simulink model "final_system"  (R2022b)
settings: Solver=FixedStepAuto  StartTime=0.0  StopTime=140  FixedStep=0.01  RelTol=1e-3
undefined symbols (not defined in the file or in its folder): heading_gain, omega0
libraries: SignalEditorBlockLib x1
settings Model: Creator=zd012  LastModifiedBy=zd012
settings DebuggingCC: UnconnectedInputMsg=warning  UnconnectedOutputMsg=warning  UnconnectedLineMsg=warning
settings ModelReferenceCC: EnableRefExpFcnMdlSchedulingChecks=on
settings RTWCC: DLArmComputeVersion=19.05

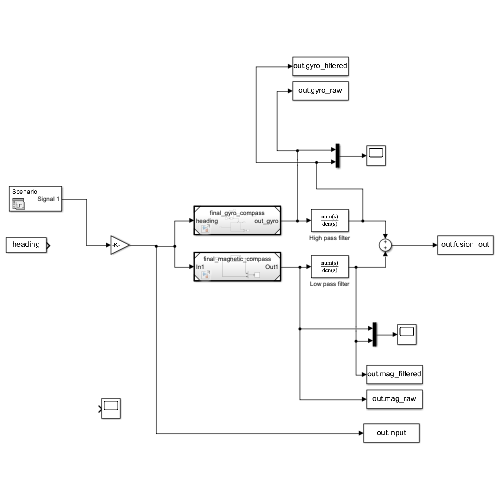
[thumbnail: Simulink's stored preview of the top-level diagram]
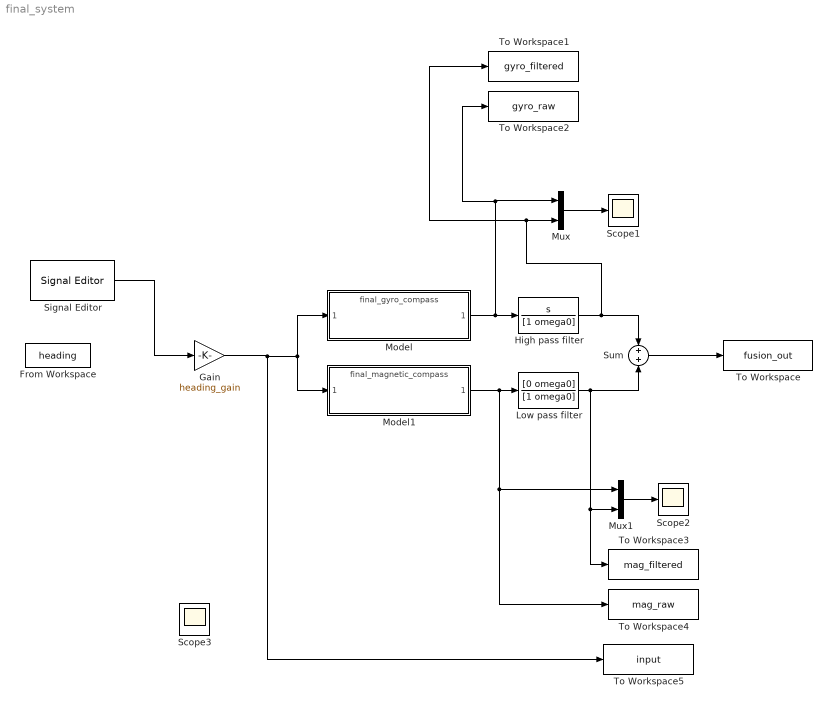
== system final_system ==
  From Workspace : FromWorkspace  VariableName=heading
  Gain : Gain  Gain=heading_gain
  High pass filter : TransferFcn  Numerator=[1 0]  Denominator=[1 omega0]
  Low pass filter : TransferFcn  Numerator=[0 omega0]  Denominator=[1 omega0]
  Model : ModelReference  ModelNameDialog=final_gyro_compass  SimulationMode=Normal  ModelReferenceVersion=4.6
  Model1 : ModelReference  ModelNameDialog=final_magnetic_compass  SimulationMode=Normal  ModelReferenceVersion=4.5
  Mux : Mux  Inputs=2
  Mux1 : Mux  Inputs=2
  Scope1 : Scope
  Scope2 : Scope
  Scope3 : Scope
  Signal Editor : SignalEditorBlockLib/Signal Editor  FileName=heading_seed.mat  ActiveScenario=Scenario  ActiveSignal=Signal 1  IsBus=off  OutputBusObjectStr=Bus: BusObject  SampleTime=0  ZeroCross=off  OutputAfterFinalValue=Setting to zero  Unit=inherit  PreserveSignalName=on
  Sum : Sum  Inputs=+|+
  To Workspace : ToWorkspace  VariableName=fusion_out  SampleTime=-1
      settings: Save2DSignal=2-D array (concatenate along first dimension)
  To Workspace1 : ToWorkspace  VariableName=gyro_filtered  SampleTime=-1
      settings: Save2DSignal=2-D array (concatenate along first dimension)
  To Workspace2 : ToWorkspace  VariableName=gyro_raw  SampleTime=-1
      settings: Save2DSignal=2-D array (concatenate along first dimension)
  To Workspace3 : ToWorkspace  VariableName=mag_filtered  SampleTime=-1
      settings: Save2DSignal=2-D array (concatenate along first dimension)
  To Workspace4 : ToWorkspace  VariableName=mag_raw  SampleTime=-1
      settings: Save2DSignal=2-D array (concatenate along first dimension)
  To Workspace5 : ToWorkspace  VariableName=input  SampleTime=-1
      settings: Save2DSignal=2-D array (concatenate along first dimension)
  wires:
  Model/1 -> To Workspace2/1, Mux/1, High pass filter/1
  High pass filter/1 -> To Workspace1/1, Mux/2, Sum/1
  Mux/1 -> Scope1/1
  Model1/1 -> To Workspace4/1, Mux1/1, Low pass filter/1
  Mux1/1 -> Scope2/1
  Low pass filter/1 -> To Workspace3/1, Mux1/2, Sum/2
  Sum/1 -> To Workspace/1
  Gain/1 -> To Workspace5/1, Model/1, Model1/1
  Signal Editor/1 -> Gain/1
